simulink model "test_TMU5KV400"  (R2018b)
settings: Solver=VariableStepAuto  StartTime=0.0  StopTime=30  RelTol=1e-3
settings Model: Creator=39926  LastModifiedBy=39926

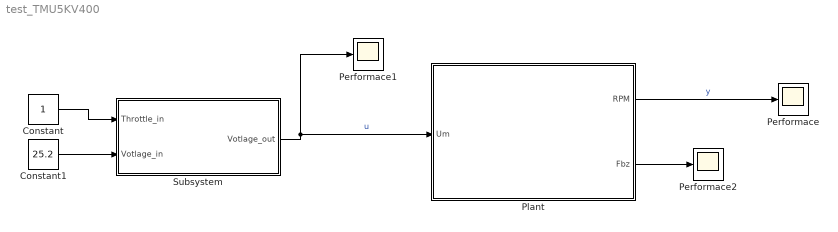
== system test_TMU5KV400 ==
  Constant : Constant
  Constant1 : Constant  Value=25.2
  Performace : Scope
  Performace1 : Scope
  Performace2 : Scope
  Plant : Subsystem
  Subsystem : Subsystem
  wires:
  Constant/1 -> Subsystem/1(Throttle_in)
  Subsystem/1(Votlage_out) -> Performace1/1, Plant/1(Um)  "u"
  Plant/1(RPM) -> Performace/1  "y"
  Plant/2("Fbz ") -> Performace2/1
  Constant1/1 -> Subsystem/2(Votlage_in)

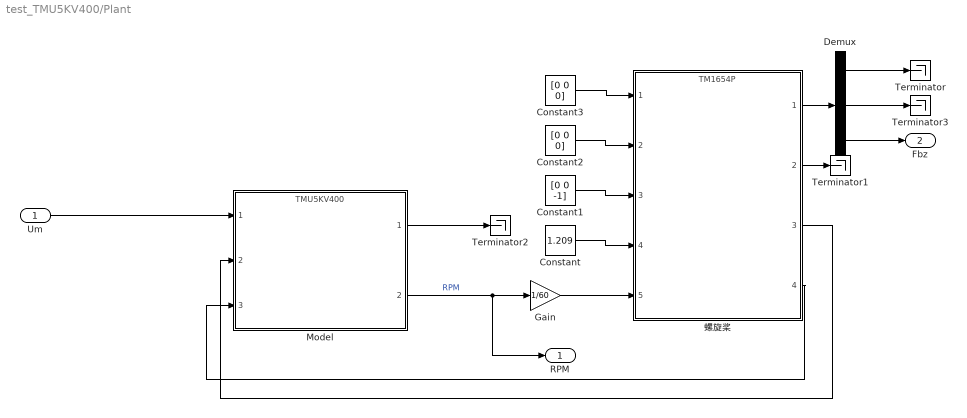
== system test_TMU5KV400/Plant ==
  Um : Inport
  Constant : Constant  Value=1.209  SampleTime=0.02
  Constant1 : Constant  Value=[0 0 -1]  SampleTime=0.02
  Constant2 : Constant  Value=[0 0 0]  SampleTime=0.02
  Constant3 : Constant  Value=[0 0 0]  SampleTime=0.02
  Demux : Demux  Outputs=3
  Gain : Gain  Gain=1/60
  Model : ModelReference  ModelNameDialog=TMU5KV400.slx  SimulationMode=Normal  ModelReferenceVersion=1.25
  Terminator{,1..3} (4 alike) : Terminator
  螺旋桨 : ModelReference  ModelNameDialog=TM1654P  SimulationMode=Normal  ModelReferenceVersion=1.90
  RPM : Outport
  "Fbz " : Outport  Port=2
  wires:
  Model/1 -> Terminator2/1
  Constant2/1 -> 螺旋桨/2
  螺旋桨/3 -> Model/2
  Constant3/1 -> 螺旋桨/1
  Model/2 -> RPM/1, Gain/1  "RPM"
  Um/1 -> Model/1
  Constant1/1 -> 螺旋桨/3
  Constant/1 -> 螺旋桨/4
  螺旋桨/4 -> Model/3
  Gain/1 -> 螺旋桨/5
  螺旋桨/1 -> Demux/1
  螺旋桨/2 -> Terminator1/1
  Demux/1 -> Terminator/1
  Demux/2 -> Terminator3/1
  Demux/3 -> "Fbz "/1

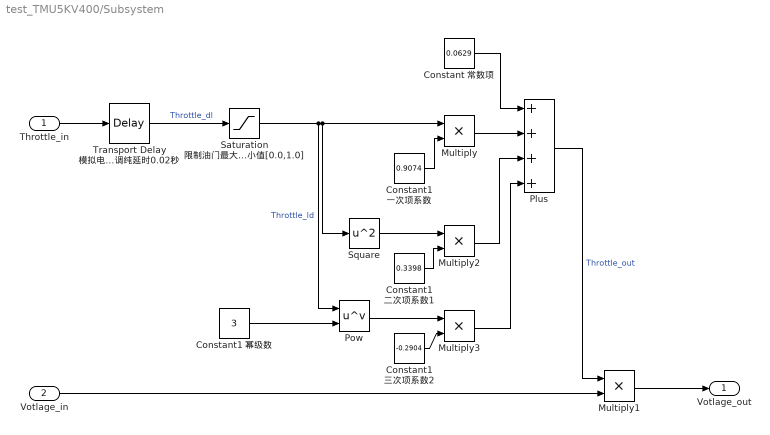
== system test_TMU5KV400/Subsystem ==
  Throttle_in : Inport  PortDimensions=1
  Votlage_in : Inport  Port=2
  Constant 常数项 : Constant  Value=0.0629
  Constant1 一次项系数 : Constant  Value=0.9074
  Constant1 三次项系数2 : Constant  Value=-0.2904
  Constant1 二次项系数1 : Constant  Value=0.3398
  Constant1 幂级数 : Constant  Value=3
  Multiply{,1..3} (4 alike) : Product
  Plus : Sum  Inputs=++++
  Pow : Math  Operator=pow  RndMeth=Zero  SaturateOnIntegerOverflow=on
  Saturation 限制油门最大最小值[0.0,1.0] : Saturate  UpperLimit=1.0  LowerLimit=0.0
  Square : Math  Operator=square  SaturateOnIntegerOverflow=on
  Transport Delay 模拟电调纯延时0.02秒 : TransportDelay  DelayTime=0.02
  Votlage_out : Outport
  wires:
  Multiply1/1 -> Votlage_out/1
  Votlage_in/1 -> Multiply1/2
  Saturation 限制油门最大最小值[0.0,1.0]/1 -> Pow/1, Square/1, Multiply/1  "Throttle_ld"
  Transport Delay 模拟电调纯延时0.02秒/1 -> Saturation 限制油门最大最小值[0.0,1.0]/1  "Throttle_dl"
  Constant1 一次项系数/1 -> Multiply/2
  Constant 常数项/1 -> Plus/1
  Multiply/1 -> Plus/2
  Multiply2/1 -> Plus/3
  Throttle_in/1 -> Transport Delay 模拟电调纯延时0.02秒/1
  Constant1 三次项系数2/1 -> Multiply3/2
  Constant1 二次项系数1/1 -> Multiply2/2
  Constant1 幂级数/1 -> Pow/2
  Square/1 -> Multiply2/1
  Pow/1 -> Multiply3/1
  Plus/1 -> Multiply1/1  "Throttle_out"
  Multiply3/1 -> Plus/4
